simulink model "admire_linear_xcs"  (Simulink 3.00)
settings: Solver=ode4  StartTime=0.0  StopTime=2  FixedStep=0.008  RelTol=1e-3
undefined symbols (not defined in the file or in its folder): Abare, Afcs, Alt, Bbare, Bfcs, Cbare, Cfcs, dasatc1_c, dasatc1_ie, dasatc1_le, dasatc1_oe, dasatc1_r, dasatc2_c, dasatc2_ie, dasatc2_le, dasatc2_oe, dasatc2_r, Dbare, ddc_bw, ddc_rate, ddei_bw, ddei_rate, ddey_bw, ddey_rate, ddle_bw, ddle_rate, ddr_bw, ddr_rate, Dfcs, Mach, rlimit_c, rlimit_ie, rlimit_le, rlimit_oe, rlimit_r, rlselect, saabgain_c, saabgain_ie, saabgain_le, saabgain_oe, saabgain_r, saabtc1_c, saabtc1_ie, saabtc1_le, saabtc1_oe, saabtc1_r, saabtc2_c, saabtc2_ie, saabtc2_le, saabtc2_oe, saabtc2_r, y0bare
libraries: simulink_extras x48
(part 2 of 2)

== system admire_linear_xcs/FCS_ae_rl/FCS_ae_rl_rie/RL3_superblock ==
  note: Level VI
  note: DASA Phase Compensating Filter
  In : Inport  Port=1  PortWidth=-1  SampleTime=-1  DataType=auto
      settings: SignalType=auto
  RL3_rie_dz : DeadZone  LowerValue=-rlimit_ie  UpperValue=rlimit_ie
  RL3_rie_rl : RateLimiter  RisingSlewLimit=rlimit_ie  FallingSlewLimit=-rlimit_ie
  RL3_rie_tf1 (with initial state) : simulink_extras/Additional Linear/Transfer Fcn (with initial states)  N=[1 0]  D=[dasatc1_ie 1]  X0=[]
  RL3_rie_tf2 (with initial state) : simulink_extras/Additional Linear/Transfer Fcn (with initial states)  N=[dasatc2_ie]  D=[dasatc2_ie 1]  X0=[]
  Sum2 : Sum  Inputs=+-  SaturateOnIntegerOverflow=on
  Out : Outport  Port=1  InitialOutput=0
  wires:
  RL3_rie_dz/1 -> RL3_rie_tf2 (with initial state)/1
  RL3_rie_tf1 (with initial state)/1 -> RL3_rie_dz/1
  In/1 -> Sum2/1, RL3_rie_tf1 (with initial state)/1
  RL3_rie_rl/1 -> Out/1
  Sum2/1 -> RL3_rie_rl/1
  RL3_rie_tf2 (with initial state)/1 -> Sum2/2

== system admire_linear_xcs/FCS_ae_rl/FCS_ae_rl_rie/RL4_superblock ==
  note: Level VI
  note: SAAB Phase Compensating Filter
  In : Inport  Port=1  PortWidth=-1  SampleTime=-1  DataType=auto
      settings: SignalType=auto
  RL4_rie__rl1 : RateLimiter  RisingSlewLimit=rlimit_ie  FallingSlewLimit=-rlimit_ie
  RL4_rie_rl2 : RateLimiter  RisingSlewLimit=rlimit_ie  FallingSlewLimit=-rlimit_ie
  RL_rie_tf1 (with initial state) : simulink_extras/Additional Linear/Transfer Fcn (with initial states)  N=[1]  D=[saabtc1_ie 1]  X0=[]
  RL_rie_tf2 (with initial state) : simulink_extras/Additional Linear/Transfer Fcn (with initial states)  Orientation=left  N=[saabgain_ie]  D=[saabtc2_ie 1]  X0=[]
  Sum24 : Sum  Inputs=-+  SaturateOnIntegerOverflow=on
  Sum25 : Sum  Inputs=-+  SaturateOnIntegerOverflow=on
  Sum26 : Sum  Inputs=+-  SaturateOnIntegerOverflow=on
  Sum27 : Sum  Inputs=++  SaturateOnIntegerOverflow=on
  Out : Outport  Port=1  InitialOutput=0
  wires:
  RL4_rie_rl2/1 -> Out/1
  Sum27/1 -> RL4_rie_rl2/1
  RL4_rie__rl1/1 -> Sum26/2, Sum27/1
  Sum25/1 -> RL4_rie__rl1/1, Sum26/1
  Sum26/1 -> RL_rie_tf2 (with initial state)/1
  Sum24/1 -> Sum27/2
  RL_rie_tf2 (with initial state)/1 -> Sum25/1
  RL_rie_tf1 (with initial state)/1 -> Sum24/1, Sum25/2
  In/1 -> Sum24/2, RL_rie_tf1 (with initial state)/1

== system admire_linear_xcs/FCS_ae_rl/FCS_ae_rl_roe/RL3_superblock ==
  note: DASA Phase Compensating Filter
  note: Level VI
  In : Inport  Port=1  PortWidth=-1  SampleTime=-1  DataType=auto
      settings: SignalType=auto
  RL3_roe_dz : DeadZone  LowerValue=-rlimit_oe  UpperValue=rlimit_oe
  RL3_roe_rl : RateLimiter  RisingSlewLimit=rlimit_oe  FallingSlewLimit=-rlimit_oe
  RL3_roe_tf1 (with initial state) : simulink_extras/Additional Linear/Transfer Fcn (with initial states)  N=[1 0]  D=[dasatc1_oe 1]  X0=[]
  RL3_roe_tf2 (with initial state) : simulink_extras/Additional Linear/Transfer Fcn (with initial states)  N=[dasatc2_oe]  D=[dasatc2_oe 1]  X0=[]
  Sum2 : Sum  Inputs=+-  SaturateOnIntegerOverflow=on
  Out : Outport  Port=1  InitialOutput=0
  wires:
  RL3_roe_tf2 (with initial state)/1 -> Sum2/2
  Sum2/1 -> RL3_roe_rl/1
  RL3_roe_rl/1 -> Out/1
  In/1 -> RL3_roe_tf1 (with initial state)/1, Sum2/1
  RL3_roe_tf1 (with initial state)/1 -> RL3_roe_dz/1
  RL3_roe_dz/1 -> RL3_roe_tf2 (with initial state)/1

== system admire_linear_xcs/FCS_ae_rl/FCS_ae_rl_roe/RL4_superblock ==
  note: SAAB Phase Compensating Filter
  note: Level VI
  In : Inport  Port=1  PortWidth=-1  SampleTime=-1  DataType=auto
      settings: SignalType=auto
  RL4_roe__rl1 : RateLimiter  RisingSlewLimit=rlimit_oe  FallingSlewLimit=-rlimit_oe
  RL4_roe_rl2 : RateLimiter  RisingSlewLimit=rlimit_oe  FallingSlewLimit=-rlimit_oe
  RL_roe_tf1 (with initial state) : simulink_extras/Additional Linear/Transfer Fcn (with initial states)  N=[1]  D=[saabtc1_oe 1]  X0=[]
  RL_roe_tf2 (with initial state) : simulink_extras/Additional Linear/Transfer Fcn (with initial states)  Orientation=left  N=[saabgain_oe]  D=[saabtc2_oe 1]  X0=[]
  Sum24 : Sum  Inputs=-+  SaturateOnIntegerOverflow=on
  Sum25 : Sum  Inputs=-+  SaturateOnIntegerOverflow=on
  Sum26 : Sum  Inputs=+-  SaturateOnIntegerOverflow=on
  Sum27 : Sum  Inputs=++  SaturateOnIntegerOverflow=on
  Out : Outport  Port=1  InitialOutput=0
  wires:
  In/1 -> RL_roe_tf1 (with initial state)/1, Sum24/2
  RL_roe_tf1 (with initial state)/1 -> Sum25/2, Sum24/1
  RL_roe_tf2 (with initial state)/1 -> Sum25/1
  Sum24/1 -> Sum27/2
  Sum26/1 -> RL_roe_tf2 (with initial state)/1
  Sum25/1 -> Sum26/1, RL4_roe__rl1/1
  RL4_roe__rl1/1 -> Sum27/1, Sum26/2
  Sum27/1 -> RL4_roe_rl2/1
  RL4_roe_rl2/1 -> Out/1
